simulink model "radio_bridge_rateChangeFilter_4x_2ch"  (Simulink 6.6)
settings: Solver=ode45  StartTime=0.0  StopTime=1e3  RelTol=1e-3
undefined symbols (not defined in the file): intfilt
libraries: xbsIndex_r4 x134
(part 2 of 2)

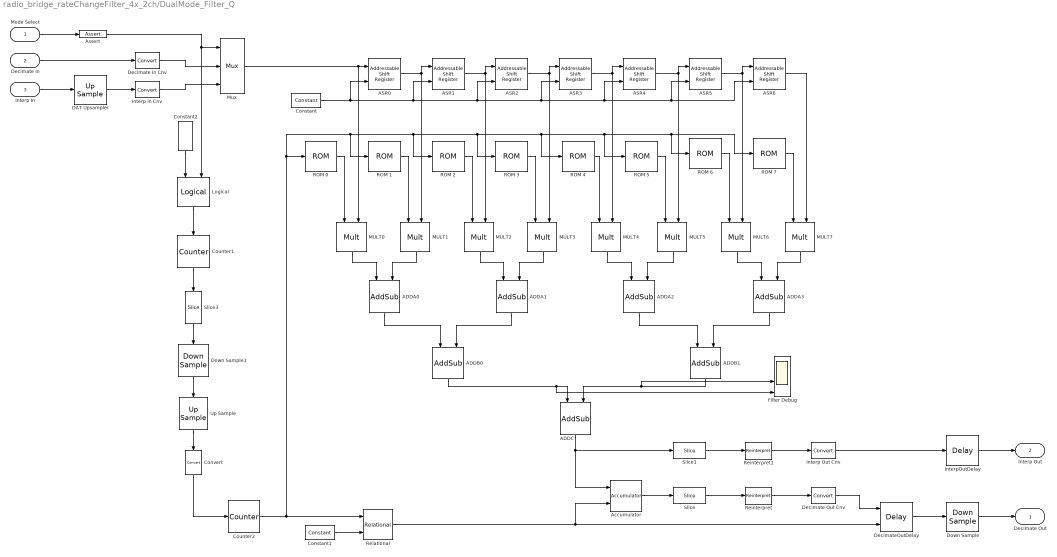
== system radio_bridge_rateChangeFilter_4x_2ch/DualMode_Filter_Q ==
  Mode Select : Inport
  Decimate In : Inport  Port=2  OutDataType=sfix(14)  OutScaling=2^-13
  Interp In : Inport  Port=3
  ADDA{0..3} (4 alike) : xbsIndex_r4/AddSub  Orientation=down  mode=Addition  use_carryin=off  use_carryout=off  en=off  latency=1  precision=Full  arith_type=Unsigned  n_bits=16  bin_pt=14  quantization=Truncate  overflow=Wrap  dbl_ovrd=off  use_behavioral_HDL=off  pipelined=off  use_rpm=on  block_type=addsub
      settings: block_version=8.2.01
  ADDB0 : xbsIndex_r4/AddSub  Orientation=down  mode=Addition  use_carryin=off  use_carryout=off  en=off  latency=1  precision=Full  arith_type=Unsigned  n_bits=16  bin_pt=14  quantization=Truncate  overflow=Wrap  dbl_ovrd=off  use_behavioral_HDL=off  pipelined=off  use_rpm=on  block_type=addsub
      settings: block_version=8.2.01
  ADDB1 : xbsIndex_r4/AddSub  Orientation=down  mode=Addition  use_carryin=off  use_carryout=off  en=off  latency=1  precision=Full  arith_type=Unsigned  n_bits=16  bin_pt=14  quantization=Truncate  overflow=Wrap  dbl_ovrd=off  use_behavioral_HDL=off  pipelined=off  use_rpm=on  block_type=addsub
      settings: block_version=8.2.01
  ADDC : xbsIndex_r4/AddSub  Orientation=down  mode=Addition  use_carryin=off  use_carryout=off  en=off  latency=1  precision=Full  arith_type="Signed  (2's comp)"  n_bits=2  bin_pt=1  quantization="Round  (unbiased: +/- Inf)"  overflow=Saturate  dbl_ovrd=off  use_behavioral_HDL=off  pipelined=off  use_rpm=on  block_type=addsub
      settings: block_version=8.2.01
  ASR{0..6} (7 alike) : xbsIndex_r4/Addressable Shift Register  infer_latency=off  depth=4  initVector=[0]  en=off  dbl_ovrd=off  use_behavioral_HDL=off  use_rpm=off  block_type=addrsr
      settings: block_version=8.2.01
      settings: infoedit=|
      | Delay of  configurable length.  Any element  in the delay
      |     line   can    be   addressed   and   driven    onto   the   output
      |     port.<P><P>Hardware  notes: Implemented  using SRL16s.
      |     If Virtex-4, Virtex-II or Spartan-3 devices are used, multiple SRLC16s are cascaded together.
  Accumulator : xbsIndex_r4/Accumulator  operation=Add  n_bits=internal_data_ibits + internal_coeff_ibits + internal_data_fbits + internal_coeff_fbits + 4  overflow=Wrap  scale=1  rst=on  hasbypass=on  en=off  dbl_ovrd=off  use_behavioral_HDL=on  block_type=accum
      settings: infoedit="Adder or subtractor-based accumulator.   Output type and binary point position match the input.<P><P>Hardware notes: When \"Reinitialize with input 'b' on reset\" is selected, the accumulator is forced to run at the system rate even if the input 'b' is running at a slower rate."  block_version=8.2.01
  Assert : xbsIndex_r4/Assert  assert_type=on  type_source=Explicitly  arith_type=Boolean  n_bits=16  bin_pt=14  assert_rate=off  rate_source=Explicitly  period=1  output_port=on  block_type=assert
      settings: infoedit=Asserts a user-defined sample rate and/or type on a signal.<P><P>Hardware notes: In hardware this block costs nothing.  block_version=10.1
  Constant : xbsIndex_r4/Constant  arith_type=Unsigned  const=3  n_bits=2  bin_pt=0  explicit_period=off  period=1  equ=P=C  opselect=C  inp2=PCIN>>17  opr=+  inp1=P  carry=CIN  dbl_ovrd=off  block_type=constant
      settings: block_version=8.2.01
  Constant1 : xbsIndex_r4/Constant  arith_type=Unsigned  const=0  n_bits=2  bin_pt=0  explicit_period=off  period=1  equ=P=C  opselect=C  inp2=PCIN>>17  opr=+  inp1=P  carry=CIN  dbl_ovrd=off  block_type=constant
      settings: block_version=8.2.01
  Constant2 : xbsIndex_r4/Constant  Orientation=down  arith_type=Boolean  const=1  n_bits=16  bin_pt=14  explicit_period=off  period=1  equ=P=C  opselect=C  inp2=PCIN>>17  opr=+  inp1=P  carry=CIN  dbl_ovrd=off  block_type=constant
      settings: block_version=8.2.01
  Convert : xbsIndex_r4/Convert  Orientation=down  arith_type=Boolean  n_bits=16  bin_pt=14  quantization=Truncate  overflow=Wrap  latency=0  dbl_ovrd=off  pipeline=off  block_type=convert
      settings: block_version=8.2.01
  Counter1 : xbsIndex_r4/Counter  Orientation=down  cnt_type=Free Running  cnt_to=Inf  operation=Up  start_count=0  cnt_by_val=1  arith_type=Unsigned  n_bits=3  bin_pt=0  load_pin=off  rst=off  en=on  explicit_period=off  period=1  dbl_ovrd=off  use_behavioral_HDL=off  use_rpm=off  block_type=counter
      settings: block_version=8.2.01
  Counter2 : xbsIndex_r4/Counter  cnt_type=Free Running  cnt_to=Inf  operation=Up  start_count=0  cnt_by_val=1  arith_type=Unsigned  n_bits=2  bin_pt=0  load_pin=off  rst=on  en=off  explicit_period=off  period=1  dbl_ovrd=off  use_behavioral_HDL=off  use_rpm=off  block_type=counter
      settings: block_version=8.2.01
  DAT Upsampler : xbsIndex_r4/Up Sample  sample_ratio=4  copy_samples=on  dbl_ovrd=off  block_type=usamp
      settings: infoedit="Up samples input data.  Inserted values  can be zeros or copies of the most recent input sample.<P><P>Hardware notes: No hardware is needed if inserted values are copies of the input sample; otherwise, a mux and single bit flip-flop are used."  block_version=8.2.01
  Decimate In Cnv : xbsIndex_r4/Convert  arith_type="Signed  (2's comp)"  n_bits=internal_data_ibits + internal_data_fbits  bin_pt=internal_data_fbits  quantization=Truncate  overflow=Wrap  latency=1  dbl_ovrd=off  pipeline=off  block_type=convert
      settings: block_version=8.2.01
  Decimate Out Cnv : xbsIndex_r4/Convert  arith_type="Signed  (2's comp)"  n_bits=decimate_out_data_width  bin_pt=decimate_out_data_bp  quantization="Round  (unbiased: +/- Inf)"  overflow=Saturate  latency=0  dbl_ovrd=off  pipeline=off  block_type=convert
      settings: block_version=8.2.01
  DecimateOutDelay : xbsIndex_r4/Delay  en=on  latency=1  dbl_ovrd=off  reg_retiming=off  block_type=delay
      settings: infoedit=Hardware notes: A delay line is a chain, each link of which is an SRL16 followed by a flip-flop. If register retiming is enabled, the delay line is a chain of flip-flops.  block_version=8.2.01
  Down Sample : xbsIndex_r4/Down Sample  sample_ratio=4  sample_phase="Last Value of Frame  (most efficient)"  en=off  latency=1  dbl_ovrd=off  block_type=dsamp
      settings: block_version=8.2.01
  Down Sample1 : xbsIndex_r4/Down Sample  Orientation=down  sample_ratio=4  sample_phase="Last Value of Frame  (most efficient)"  en=off  latency=1  dbl_ovrd=off  block_type=dsamp
      settings: block_version=8.2.01
  Filter Debug : Scope  NumInputPorts=4
      settings: TickLabels=on  TimeRange=1000  YMin=-1~-1~-1~-1  YMax=1~1~1~1  SaveName=ScopeData2
  Interp In Cnv : xbsIndex_r4/Convert  arith_type="Signed  (2's comp)"  n_bits=internal_data_ibits + internal_data_fbits  bin_pt=internal_data_fbits  quantization=Truncate  overflow=Wrap  latency=1  dbl_ovrd=off  pipeline=off  block_type=convert
      settings: block_version=8.2.01
  Interp Out Cnv : xbsIndex_r4/Convert  arith_type="Signed  (2's comp)"  n_bits=interp_out_data_width  bin_pt=interp_out_data_bp  quantization="Round  (unbiased: +/- Inf)"  overflow=Saturate  latency=0  dbl_ovrd=off  pipeline=off  block_type=convert
      settings: block_version=8.2.01
  InterpOutDelay : xbsIndex_r4/Delay  en=off  latency=1  dbl_ovrd=off  reg_retiming=off  block_type=delay
      settings: infoedit=Hardware notes: A delay line is a chain, each link of which is an SRL16 followed by a flip-flop. If register retiming is enabled, the delay line is a chain of flip-flops.  block_version=8.2.01
  Logical : xbsIndex_r4/Logical  Orientation=down  logical_function=OR  inputs=2  en=off  latency=0  precision=Full  arith_type=Unsigned  n_bits=16  bin_pt=0  align_bp=on  dbl_ovrd=off  block_type=logical
      settings: block_version=8.2.01
  MULT{0..7} (8 alike) : xbsIndex_r4/Mult  Orientation=down  precision=Full  arith_type="Signed  (2's comp)"  n_bits=16  bin_pt=14  quantization=Truncate  overflow=Wrap  en=off  latency=1  dbl_ovrd=off  use_behavioral_HDL=off  use_embedded=on  opt=Speed  optimum_pipeline=off  pipeline=on  use_rpm=on  placement_style=Rectangular shape  block_type=mult
      settings: infoedit=Hardware notes: To use the internal pipeline stage of the dedicated multiplier you must select 'Pipeline for maximum performance'.  block_version=8.2.01
  Mux : xbsIndex_r4/Mux  inputs=2  en=off  latency=1  precision=Full  arith_type=Unsigned  n_bits=16  bin_pt=14  quantization=Truncate  overflow=Wrap  dbl_ovrd=off  block_type=mux
      settings: block_version=8.2.01
  ROM 0 : xbsIndex_r4/ROM  depth=4  initVector=[h(1:4)]  distributed_mem=Distributed memory  rst=off  init_reg=0  en=off  latency=1  arith_type="Signed  (2's comp)"  n_bits=internal_coeff_ibits + internal_coeff_fbits  bin_pt=internal_coeff_fbits  dbl_ovrd=off  optimize=Area  use_rpm=on  block_type=sprom
      settings: block_version=8.2.01
  ROM 1 : xbsIndex_r4/ROM  depth=4  initVector=[h(5:8)]  distributed_mem=Distributed memory  rst=off  init_reg=0  en=off  latency=1  arith_type="Signed  (2's comp)"  n_bits=internal_coeff_ibits + internal_coeff_fbits  bin_pt=internal_coeff_fbits  dbl_ovrd=off  optimize=Area  use_rpm=on  block_type=sprom
      settings: block_version=8.2.01
  ROM 2 : xbsIndex_r4/ROM  depth=4  initVector=[h(9:12)]  distributed_mem=Distributed memory  rst=off  init_reg=0  en=off  latency=1  arith_type="Signed  (2's comp)"  n_bits=internal_coeff_ibits + internal_coeff_fbits  bin_pt=internal_coeff_fbits  dbl_ovrd=off  optimize=Area  use_rpm=on  block_type=sprom
      settings: block_version=8.2.01
  ROM 3 : xbsIndex_r4/ROM  depth=4  initVector=[h(13:16)]  distributed_mem=Distributed memory  rst=off  init_reg=0  en=off  latency=1  arith_type="Signed  (2's comp)"  n_bits=internal_coeff_ibits + internal_coeff_fbits  bin_pt=internal_coeff_fbits  dbl_ovrd=off  optimize=Area  use_rpm=on  block_type=sprom
      settings: block_version=8.2.01
  ROM 4 : xbsIndex_r4/ROM  depth=4  initVector=[h(17:20)]  distributed_mem=Distributed memory  rst=off  init_reg=0  en=off  latency=1  arith_type="Signed  (2's comp)"  n_bits=internal_coeff_ibits + internal_coeff_fbits  bin_pt=internal_coeff_fbits  dbl_ovrd=off  optimize=Area  use_rpm=on  block_type=sprom
      settings: block_version=8.2.01
  ROM 5 : xbsIndex_r4/ROM  depth=4  initVector=[h(21:24)]  distributed_mem=Distributed memory  rst=off  init_reg=0  en=off  latency=1  arith_type="Signed  (2's comp)"  n_bits=internal_coeff_ibits + internal_coeff_fbits  bin_pt=internal_coeff_fbits  dbl_ovrd=off  optimize=Area  use_rpm=on  block_type=sprom
      settings: block_version=8.2.01
  ROM 6 : xbsIndex_r4/ROM  depth=4  initVector=[h(25:28)]  distributed_mem=Distributed memory  rst=off  init_reg=0  en=off  latency=1  arith_type="Signed  (2's comp)"  n_bits=internal_coeff_ibits + internal_coeff_fbits  bin_pt=internal_coeff_fbits  dbl_ovrd=off  optimize=Area  use_rpm=on  block_type=sprom
      settings: block_version=8.2.01
  ROM 7 : xbsIndex_r4/ROM  depth=4  initVector=[h(29:32)]  distributed_mem=Distributed memory  rst=off  init_reg=0  en=off  latency=1  arith_type="Signed  (2's comp)"  n_bits=internal_coeff_ibits + internal_coeff_fbits  bin_pt=internal_coeff_fbits  dbl_ovrd=off  optimize=Area  use_rpm=on  block_type=sprom
      settings: block_version=8.2.01
  Reinterpret : xbsIndex_r4/Reinterpret  force_arith_type=on  arith_type="Signed  (2's comp)"  force_bin_pt=on  bin_pt=decimate_out_fbits+4  block_type=reinterpret
      settings: infoedit="Changes signal type without altering the binary representation.   You can changed the signal between signed and unsigned, and relocate the binary point.<P><P>Hardware notes: In hardware this block costs nothing.<P><P>Example:  Suppose the input is 6 bits wide, signed, with 2 fractional bits, and the output is forced to unsigned with 0 fractional bits.  Then an input of -2.0 (1110.00 in binary 2's complement) becomes an output of 56 (111000 in binary)."  block_version=8.2.01
  Reinterpret1 : xbsIndex_r4/Reinterpret  force_arith_type=on  arith_type="Signed  (2's comp)"  force_bin_pt=on  bin_pt=interp_out_fbits+4  block_type=reinterpret
      settings: infoedit="Changes signal type without altering the binary representation.   You can changed the signal between signed and unsigned, and relocate the binary point.<P><P>Hardware notes: In hardware this block costs nothing.<P><P>Example:  Suppose the input is 6 bits wide, signed, with 2 fractional bits, and the output is forced to unsigned with 0 fractional bits.  Then an input of -2.0 (1110.00 in binary 2's complement) becomes an output of 56 (111000 in binary)."  block_version=8.2.01
  Relational : xbsIndex_r4/Relational  mode=a=b  en=off  latency=1  dbl_ovrd=off  block_type=relational
      settings: block_version=8.2.01
  Slice : xbsIndex_r4/Slice  nbits=(1 + decimate_out_ibits) + (decimate_out_fbits + 4)  boolean_output=off  mode=Lower Bit Location + Width  bit1=0  base1=MSB of Input  bit0=internal_data_fbits + internal_coeff_fbits - (decimate_out_fbits + 4) + 2  base0=LSB of Input  dbl_ovrd=off  block_type=slice
      settings: infoedit="Extracts a given range of bits from each input sample and presents it at the output.  The output type is ordinarily unsigned with binary point at zero, but can be Boolean when the slice is one bit wide.<P><P>Hardware notes: In hardware this block costs nothing."  block_version=8.2.01
  Slice1 : xbsIndex_r4/Slice  nbits=(1 + interp_out_ibits) + (interp_out_fbits + 4)  boolean_output=off  mode=Lower Bit Location + Width  bit1=0  base1=MSB of Input  bit0=internal_data_fbits + internal_coeff_fbits - (interp_out_fbits + 4)  base0=LSB of Input  dbl_ovrd=off  block_type=slice
      settings: infoedit="Extracts a given range of bits from each input sample and presents it at the output.  The output type is ordinarily unsigned with binary point at zero, but can be Boolean when the slice is one bit wide.<P><P>Hardware notes: In hardware this block costs nothing."  block_version=8.2.01
  Slice3 : xbsIndex_r4/Slice  Orientation=down  nbits=1  boolean_output=off  mode=Upper Bit Location + Width  bit1=0  base1=MSB of Input  bit0=0  base0=LSB of Input  dbl_ovrd=off  block_type=slice
      settings: infoedit="Extracts a given range of bits from each input sample and presents it at the output.  The output type is ordinarily unsigned with binary point at zero, but can be Boolean when the slice is one bit wide.<P><P>Hardware notes: In hardware this block costs nothing."  block_version=8.2.01
  Up Sample : xbsIndex_r4/Up Sample  Orientation=down  sample_ratio=4  copy_samples=off  dbl_ovrd=off  block_type=usamp
      settings: infoedit="Up samples input data.  Inserted values  can be zeros or copies of the most recent input sample.<P><P>Hardware notes: No hardware is needed if inserted values are copies of the input sample; otherwise, a mux and single bit flip-flop are used."  block_version=8.2.01
  Decimate Out : Outport
  Interp Out : Outport  Port=2
  wires:
  Convert/1 -> Counter2/1
  Counter2/1 -> ROM 0/1, ROM 7/1, ROM 6/1, ROM 5/1, ROM 4/1, ROM 3/1, ROM 2/1, ROM 1/1, Relational/1
  Relational/1 -> DecimateOutDelay/2, Accumulator/2
  Constant1/1 -> Relational/2
  Up Sample/1 -> Convert/1
  Down Sample1/1 -> Up Sample/1
  Slice3/1 -> Down Sample1/1
  Counter1/1 -> Slice3/1
  Logical/1 -> Counter1/1
  Constant2/1 -> Logical/1
  Reinterpret1/1 -> Interp Out Cnv/1
  Slice1/1 -> Reinterpret1/1
  Reinterpret/1 -> Decimate Out Cnv/1
  Slice/1 -> Reinterpret/1
  Accumulator/1 -> Slice/1
  InterpOutDelay/1 -> Interp Out/1
  Mode Select/1 -> Assert/1
  Mux/1 -> MULT0/2, ASR0/1
  Interp In Cnv/1 -> Mux/3
  Decimate In Cnv/1 -> Mux/2
  DAT Upsampler/1 -> Interp In Cnv/1
  Decimate In/1 -> Decimate In Cnv/1
  Decimate Out Cnv/1 -> DecimateOutDelay/1
  Interp Out Cnv/1 -> InterpOutDelay/1
  ADDC/1 -> Slice1/1, Accumulator/1
  Interp In/1 -> DAT Upsampler/1
  Down Sample/1 -> Decimate Out/1
  ADDB1/1 -> ADDC/2, Filter Debug/3
  ADDB0/1 -> ADDC/1, Filter Debug/4
  ADDA3/1 -> ADDB1/2
  ADDA2/1 -> ADDB1/1
  ADDA1/1 -> ADDB0/2
  ADDA0/1 -> ADDB0/1
  MULT7/1 -> ADDA3/2
  MULT6/1 -> ADDA3/1
  MULT5/1 -> ADDA2/2
  MULT4/1 -> ADDA2/1
  MULT3/1 -> ADDA1/2
  MULT2/1 -> ADDA1/1
  MULT1/1 -> ADDA0/2
  MULT0/1 -> ADDA0/1
  ROM 6/1 -> MULT6/1
  ROM 5/1 -> MULT5/1
  ROM 4/1 -> MULT4/1
  ROM 3/1 -> MULT3/1
  ROM 2/1 -> MULT2/1
  ROM 7/1 -> MULT7/1
  ASR6/1 -> MULT7/2
  ROM 1/1 -> MULT1/1
  ROM 0/1 -> MULT0/1
  ASR5/1 -> MULT6/2, ASR6/1
  ASR4/1 -> MULT5/2, ASR5/1
  ASR3/1 -> MULT4/2, ASR4/1
  ASR2/1 -> MULT3/2, ASR3/1
  ASR1/1 -> MULT2/2, ASR2/1
  Constant/1 -> ASR0/2, ASR6/2, ASR5/2, ASR4/2, ASR3/2, ASR2/2, ASR1/2
  ASR0/1 -> MULT1/2, ASR1/1
  DecimateOutDelay/1 -> Down Sample/1
  Assert/1 -> Logical/2, Mux/1
